simulink model "task4"  (R2023a)
settings: Solver=VariableStepAuto  StartTime=0.0  StopTime=10.0  RelTol=1e-3
settings Model: Creator=LENOVO  LastModifiedBy=LENOVO

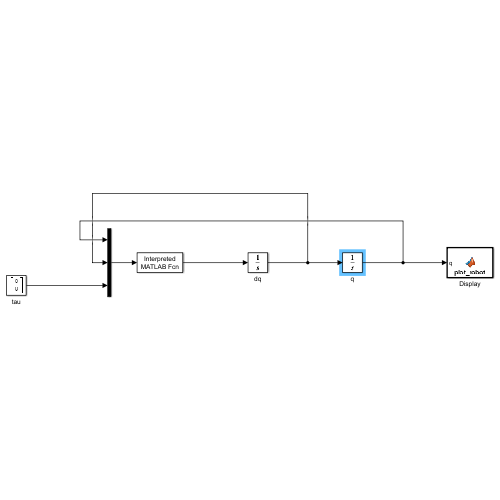
[thumbnail: Simulink's stored preview of the top-level diagram]
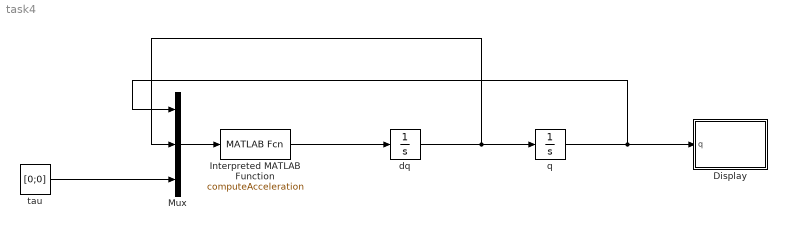
== system task4 ==
  Display : MATLAB Function  TreatAsAtomicUnit=on
  Interpreted MATLAB Function : MATLABFcn  MATLABFcn=computeAcceleration  OutputDimensions=2  Output1D=off
  Mux : Mux  Inputs=3
  dq : Integrator  InitialCondition=[0; 0]
  q : Integrator  InitialCondition=[pi; pi/2]
  tau : Constant  Value=[0;0]  VectorParams1D=off
  wires:
  dq/1 -> Mux/2, q/1
  q/1 -> Mux/1, Display/1(q)
  Interpreted MATLAB Function/1 -> dq/1
  tau/1 -> Mux/3
  Mux/1 -> Interpreted MATLAB Function/1

== matlab function task4/Display ==
  settings: updateMethod=DISCRETE
  data: q input
function plot_robot(q)
    % Persistent variables to store joint trajectories
    persistent joint1_trail joint2_trail;

    % Link lengths
    q1 = q(1);
    q2 = q(2);
    l1 = 0.3; 
    l2 = 0.2;

    % Joint positions
    x1 = l1 * cos(q1);
    y1 = l1 * sin(q1);
    x2 = x1 + l2 * cos(q1 + q2);
    y2 = y1 + l2 * sin(q1 + q2);

    % Initialize persistent variables on the first call
    if isempty(joint1_trail) || isempty(joint2_trail)
        joint1_trail = [x1, y1]; % Start at the first joint
        joint2_trail = [x2, y2]; % Start at the second joint (end effector)
    else
        % Update trails
        joint1_trail = [joint1_trail; x1, y1];
        joint2_trail = [joint2_trail; x2, y2];
    end

    % Plot the robot and its trajectory
    clf; hold on;

    % Plot the trajectory trails
    plot(joint1_trail(:, 1), joint1_trail(:, 2), 'r--', 'LineWidth', 1.5, 'DisplayName', 'Joint 1 Trajectory');
    plot(joint2_trail(:, 1), joint2_trail(:, 2), 'b--', 'LineWidth', 1.5, 'DisplayName', 'Joint 2 Trajectory');

    % Plot the robot links
    plot([0, x1, x2], [0, y1, y2], '-ko', 'LineWidth', 2, 'MarkerFaceColor', 'k', 'DisplayName', 'Robot Configuration');

    % Set plot limits and labels
    xlim([-0.6, 0.6]);
    ylim([-0.6, 0.6]);
    grid on;
    xlabel('X Position (m)');
    ylabel('Y Position (m)');
    title('Robot Trajectory and Configuration');
    legend('Location', 'best');

    % Draw the plot
    drawnow;
end
